simulink model "acc"  (R2021b)
settings: Solver=FixedStepAuto  StartTime=0.0  StopTime=206  FixedStep=0.0005  RelTol=1e-3
values from neighbouring files (symbols this model uses):
  Leftdis_PV_switch = 2    [acc_plot_backup.m]
  s_path = [0 1.10508939428 2.2141958029 3.32141571172 4.42705301151 5.53154548532 6.63517443471 7.73808041313 8.84055018688 9.94289959674 11.0453539299 12.1480581097 ... (1001 elements, 1001x1)]    [200_100radius.mat]    (also in LV_Clothoid_S_Turn_path.mat = [0 0.966832089581 1.93621320584 2.90214024471 3.86476766313 ; NEDC_path.mat = [0 0.414605943146 0.832514087334 1.25401518562 1.68216660344; Straight_East_into_curve.mat = [0 1.65770560069 3.32192925577 4.98420060507 6.64484613518 8; acc_plot_backup.m = Station_HV_m)
  X_path = [0 1.10508939428 2.2141958029 3.32141571172 4.42705301151 5.53154548532 6.63517443471 7.73808041313 8.84055018688 9.94289959674 11.0453539299 12.1480581097 ... (1001 elements, 1001x1)]    [200_100radius.mat]    (also in LV_Clothoid_S_Turn_path.mat = [-10 -9.03316791042 -8.06378679416 -7.09785975529 -6.1352323; NEDC_path.mat = [0 0.414605943146 0.832514087334 1.25401518562 1.68216660344; Straight_East_into_curve.mat = [0 1.65770560069 3.32192925577 4.98420060507 6.64484613518 8; acc_plot_backup.m = X_HV_m)
  Y_path = [0 -1.70364610795e-18 -7.41532896709e-18 1.46822109542e-17 4.74557362791e-17 6.12980216762e-17 9.25043977736e-17 1.24088240159e-16 1.5099156923e-16 1.7058517853e-16 1.90629227614e-16 2.09673434424e-16 ... (1001 elements, 1001x1)]    [200_100radius.mat]    (also in LV_Clothoid_S_Turn_path.mat = [0 -8.46153035536e-19 5.07382551045e-18 2.07356032218e-17 3.; NEDC_path.mat = [0 -3.50680326162e-18 -2.14111304971e-18 3.38197671014e-18 3; Straight_East_into_curve.mat = [0 1.29197709199e-18 2.81882429322e-18 3.49020462564e-17 6.7; acc_plot_backup.m = Y_HV_m)
undefined symbols (not defined in the file or in its folder): C_TICK_TIME_S, ENUM_ACCSTATE_DISABLED, ENUM_ACCSTATE_OFF, ENUM_ACCSTATE_STANDBY, FALSE, KVDI_ACCLongPressTime_ms, KVDI_ACCMaxActSpeed_kph, KVDI_ACCSetSpdIntial_kph, KVDI_ACCSpdLargeChange_kph, KVDI_LongPressConTime_ms, ONE_FLOAT, ONE_INT, R, Rw, T, TRUE, ZERO_FLOAT, ZERO_INT
libraries: simulink x16, dspstat3 x4, simulink_extras x2, Solver_SF x1
(part 3 of 4)

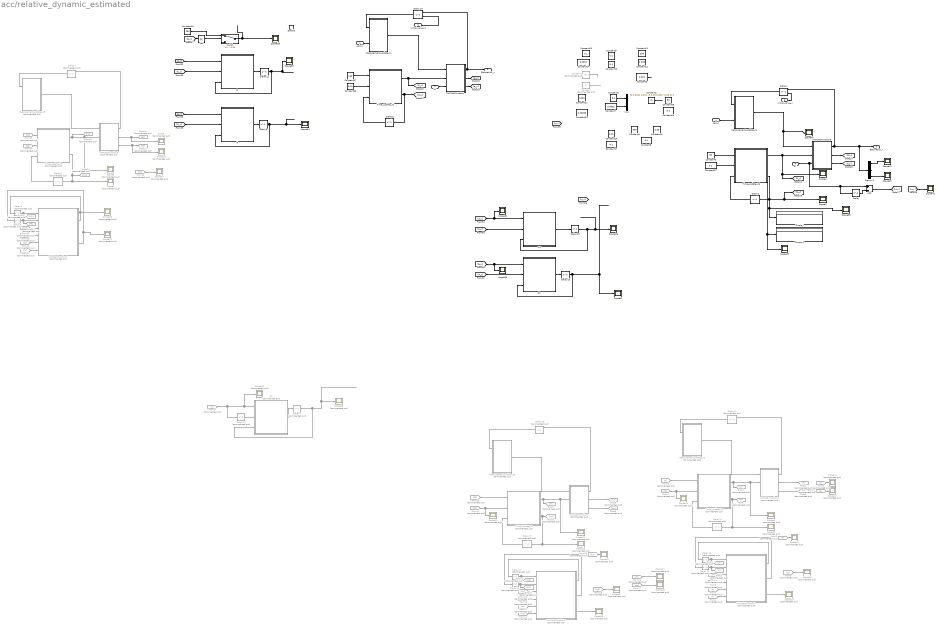
== system acc/relative_dynamic_estimated ==
  Jerk_X : Inport
  RX : Inport  Port=2
  Initial_value_X : Inport  Port=3
  Jerk_Y : Inport  Port=4
  RY : Inport  Port=5
  Initial_value_Y : Inport  Port=6
  Enable : EnablePort
  Abs : Abs
  Add : Sum  Inputs=+-
  Constant : Constant  Commented=on  Value=R
  Constant1 : Constant  Commented=on  Value=Rw
  Constant{4..5,9..10,13,17,22,24} (8 alike) : Constant  Value=0.1
  Constant11 : Constant  Value=200
  Constant12 : Constant  Value=0.005
  Constant14 : Constant  Value=0.0001
  Constant15 : Constant  Value=0.05
  Constant16 : Constant  Value=300
  Constant19 : Constant  Value=0.01
  Constant2 : Constant  Value=[0 0.0001 0.0017;0.0001 0.0025 0.05;0.0017 0.05 1]*1
  Constant20 : Constant  Value=0.00005
  Constant21 : Constant  Value=1000
  Constant25 : Constant  Value=50
  Constant26 : Constant  Value=0.01
  Constant27 : Constant  Value=100
  Constant3 : Constant  Value=0.001
  Constant6 : Constant  Value=50
  Constant7 : Constant  Value=0.0001
  Constant8 : Constant  Value=500
  Delay : Delay  DelayLength=1
  Delay1 : Delay  DelayLength=1  InitialConditionSource=Input port  InitialCondition=[0;0;0]  SampleTime=T
      settings: InputPortMap=u0,p4
  Delay10 : Delay  DelayLength=1  InitialConditionSource=Input port  InitialCondition=[0;0;0]  SampleTime=T
      settings: InputPortMap=u0,p4
  Delay11 : Delay  Commented=on  DelayLength=1  InitialConditionSource=Input port  InitialCondition=[0;0;0]  SampleTime=T
      settings: InputPortMap=u0,p4
  Delay12 : Delay  Commented=on  DelayLength=1  InitialCondition=[0 0 0;0 0 0.004;0 0.004 0.8]*0.001  SampleTime=T
  Delay13 : Delay  Commented=on  DelayLength=1  InitialCondition=0.001  SampleTime=T
  Delay14 : Delay  Commented=on  DelayLength=1  InitialCondition=[1 0 0;0 1 0;0 0 1]  SampleTime=T
  Delay15 : Delay  Commented=on  DelayLength=1  InitialConditionSource=Input port  InitialCondition=[0;0;0]  SampleTime=T
      settings: InputPortMap=u0,p4
  Delay16 : Delay  Commented=on  DelayLength=1  InitialCondition=0
  Delay17 : Delay  Commented=on  DelayLength=1  InitialCondition=[0 0 0;0 0 0.004;0 0.004 0.8]*0.01  SampleTime=T
  Delay18 : Delay  Commented=on  DelayLength=1  InitialCondition=0.001  SampleTime=T
  Delay19 : Delay  Commented=on  DelayLength=1  InitialCondition=[1 0 0;0 1 0;0 0 1]  SampleTime=T
  Delay2 : Delay  DelayLength=1  InitialCondition=[1 0 0;0 1 0;0 0 1]  SampleTime=T
  Delay21 : Delay  DelayLength=1  InitialCondition=[0 0.0001 0.0017;0.0001 0.0025 0.05;0.0017 0.05 1]
  Delay22 : Delay  DelayLength=1  InitialCondition=0.001
  Delay23 : Delay  DelayLength=1  InitialCondition=[0 0.0001 0.0017;0.0001 0.0025 0.05;0.0017 0.05 1]*1e-5
  Delay3 : Delay  Commented=on  DelayLength=1  InitialCondition=[0 0 0;0 0 0.003;0 0.003 0.005]  SampleTime=T
  Delay4 : Delay  Commented=on  DelayLength=1  InitialConditionSource=Input port  InitialCondition=[0;0;0]  SampleTime=T
      settings: InputPortMap=u0,p4
  Delay5 : Delay  Commented=on  DelayLength=1  InitialCondition=0.001  SampleTime=T
  Delay6 : Delay  Commented=on  DelayLength=1  InitialCondition=[1 0 0;0 1 0;0 0 1]  SampleTime=T
  Delay7 : Delay  Commented=on  DelayLength=1  InitialCondition=0.1
  Delay8 : Delay  DelayLength=1  InitialCondition=0.1
  Delay9 : Delay  DelayLength=1  InitialCondition=[1 0 0;0 1 0;0 0 1]  SampleTime=T
  Demux1 : Demux  Outputs=3
  Display : Display
  Display1 : Display
  From : From  Commented=on  GotoTag=M
  From1 : From  Commented=on  GotoTag=K
  From10 : From  Commented=on  GotoTag=MM
  From11 : From  Commented=on  GotoTag=KK
  From12 : From  Commented=on  GotoTag=dd
  From13 : From  Commented=on  GotoTag=ee
  From14 : From  Commented=on  GotoTag=QQ
  From15 : From  Commented=on  GotoTag=RR
  From16 : From  Commented=on  GotoTag=dd
  From17 : From  Commented=on  GotoTag=ee
  From18 : From  Commented=on  GotoTag=RR
  From19 : From  Commented=on  GotoTag=QQ
  From2 : From  Commented=on  GotoTag=d
  From20 : From  Commented=on  GotoTag=MM
  From21 : From  Commented=on  GotoTag=KK
  From22 : From  Commented=on  GotoTag=dd
  From23 : From  Commented=on  GotoTag=ee
  From24 : From  Commented=on  GotoTag=QQ
  From25 : From  Commented=on  GotoTag=RR
  From26 : From  Commented=on  GotoTag=KK
  From27 : From  Commented=on  GotoTag=d
  From3 : From  Commented=on  GotoTag=e
  From4 : From  Commented=on  GotoTag=Q
  From5 : From  Commented=on  GotoTag=R
  From6 : From  Commented=on  GotoTag=d
  From7 : From  Commented=on  GotoTag=e
  From8 : From  Commented=on  GotoTag=R
  From9 : From  Commented=on  GotoTag=Q
  Goto : Goto  Commented=on  GotoTag=M
  Goto1 : Goto  Commented=on  GotoTag=K
  Goto10 : Goto  Commented=on  GotoTag=QQ
  Goto11 : Goto  Commented=on  GotoTag=RR
  Goto12 : Goto  Commented=on  GotoTag=QQ
  Goto13 : Goto  Commented=on  GotoTag=RR
  Goto14 : Goto  Commented=on  GotoTag=MM
  Goto15 : Goto  Commented=on  GotoTag=KK
  Goto16 : Goto  Commented=on  GotoTag=dd
  Goto17 : Goto  Commented=on  GotoTag=ee
  Goto2 : Goto  Commented=on  GotoTag=d
  Goto3 : Goto  Commented=on  GotoTag=e
  Goto4 : Goto  Commented=on  GotoTag=Q
  Goto5 : Goto  Commented=on  GotoTag=R
  Goto6 : Goto  Commented=on  GotoTag=MM
  Goto7 : Goto  Commented=on  GotoTag=KK
  Goto8 : Goto  Commented=on  GotoTag=dd
  Goto9 : Goto  Commented=on  GotoTag=ee
  MATLAB Function : MATLAB Function  TreatAsAtomicUnit=on
  MATLAB Function1 : MATLAB Function  Commented=on  TreatAsAtomicUnit=on
  MATLAB Function2 : MATLAB Function  Commented=on  TreatAsAtomicUnit=on
  MATLAB Function3 : MATLAB Function  Commented=on  TreatAsAtomicUnit=on
  MATLAB Function4 : MATLAB Function  Commented=on  TreatAsAtomicUnit=on
  MATLAB Function5 : MATLAB Function  TreatAsAtomicUnit=on
  MATLAB Function6 : MATLAB Function  Commented=on  TreatAsAtomicUnit=on
  MATLAB Function7 : MATLAB Function  Commented=on  TreatAsAtomicUnit=on
  Measurement_update_X1 : MATLAB Function  TreatAsAtomicUnit=on
  Measurement_update_X2 : MATLAB Function  Commented=on  TreatAsAtomicUnit=on
  Measurement_update_X3 : MATLAB Function  Commented=on  TreatAsAtomicUnit=on
  Measurement_update_X4 : MATLAB Function  TreatAsAtomicUnit=on
  Measurement_update_X5 : MATLAB Function  Commented=on  TreatAsAtomicUnit=on
  Mux : Mux  Inputs=2
  Q : MATLAB Function  TreatAsAtomicUnit=on
  Q1 : MATLAB Function  Commented=on  TreatAsAtomicUnit=on
  Q2 : MATLAB Function  TreatAsAtomicUnit=on
  R : MATLAB Function  TreatAsAtomicUnit=on
  R2 : MATLAB Function  TreatAsAtomicUnit=on
  Scope{,6..28,30} (25 alike) : Scope  Commented=on
  Scope{1..2,5,29,31,34..43} (15 alike) : Scope
  Switch : Switch  Criteria=u2 > Threshold  Threshold=0.04
  Time_update_X1 : MATLAB Function  TreatAsAtomicUnit=on
  Time_update_X2 : MATLAB Function  Commented=on  TreatAsAtomicUnit=on
  Time_update_X3 : MATLAB Function  Commented=on  TreatAsAtomicUnit=on
  Time_update_X5 : MATLAB Function  Commented=on  TreatAsAtomicUnit=on
  Time_update_X6 : MATLAB Function  TreatAsAtomicUnit=on
  Estimation_X : Outport  VectorParamsAs1DForOutWhenUnconnected=off
  Estimation_Y : Outport  Port=2  VectorParamsAs1DForOutWhenUnconnected=off
  wires:
  MATLAB Function/3(e) -> [e_x]
  MATLAB Function/2(d) -> [d_x]
  Constant27/1 -> Time_update_X1/1(Q)
  Constant26/1 -> Time_update_X1/2(R)
  Abs/1 -> Switch/2
  [d_x] -> Abs/1
  Constant16/1 -> Switch/1
  Switch/1 -> Scope39/1
  Constant22/1 -> Time_update_X6/2(R)
  Constant6/1 -> Time_update_X6/1(Q)
  Demux1/3 -> Scope43/1
  Demux1/1 -> Scope42/1
  [yyy] -> Scope41/1
  Delay/1 -> Add/2
  Add/1 -> [yyy]
  Delay22/1 -> Scope5/1, R2/3(R1)
  Constant7/1 -> Mux/2
  Constant4/1 -> Mux/1
  Demux1/2 -> ?
  Delay23/1 -> Scope36/1, Q2/3(Q1)
  Time_update_X6/2(P) -> Display1/1, Scope37/1
  Constant3/1 -> ?
  Constant2/1 -> ?
  Q2/1(Q) -> Delay23/1
  Constant1/1 -> ?
  Constant/1 -> ?
  MATLAB Function5/3(e) -> [e_y]
  MATLAB Function5/2(d) -> [d_y]
  [d_y] -> Q2/1(d), Scope31/1
  [K_y] -> Q2/2(K)
  R2/1(R) -> Delay22/1
  [M_y] -> R2/2(M)
  [e_y] -> R2/1(e), Scope29/1
  Q1/1(Rw) -> Delay7/1
  From27/1 -> Q1/1(d), Scope30/1, Delay16/1
  Delay7/1 -> Scope28/1, Q1/3(Rw1)
  Delay16/1 -> Q1/2(dx)
  Delay21/1 -> Q/3(Q1), Scope35/1
  Q/1(Q) -> Delay21/1
  [K_x] -> Q/2(K)
  [d_x] -> Q/1(d)
  [M_x] -> R/2(M)
  R/1(R) -> Delay8/1
  [e_x] -> R/1(e)
  Delay8/1 -> R/3(R1), Scope34/1
  RX/1 -> MATLAB Function/3(y)
  From26/1 -> Scope27/1
  Initial_value_X/1 -> Delay10/2
  Delay4/1 -> Measurement_update_X5/1(X_e)
  MATLAB Function6/1(X_e) -> Delay4/1
  Measurement_update_X5/1(X_b) -> MATLAB Function6/1(X_b)
  Time_update_X5/2(M2) -> Scope7/1, Delay6/1, Goto14/1
  From22/1 -> MATLAB Function7/5(d)
  Delay6/1 -> Time_update_X5/3(M)
  Time_update_X5/1(K) -> MATLAB Function6/2(K), Scope6/1, Goto15/1
  From21/1 -> MATLAB Function7/6(K)
  From20/1 -> MATLAB Function7/3(M)
  MATLAB Function7/2(R2) -> Delay5/1, Scope26/1
  MATLAB Function6/3(e) -> Goto17/1, Scope24/1
  From24/1 -> Time_update_X5/2(Q)
  From25/1 -> Time_update_X5/1(R)
  MATLAB Function7/1(Q2) -> Scope25/1, Delay3/1
  From23/1 -> MATLAB Function7/4(e)
  Delay5/1 -> Goto13/1, MATLAB Function7/2(R)
  Delay3/1 -> Goto12/1, MATLAB Function7/1(Q)
  MATLAB Function6/2(d) -> Goto16/1, Scope/1
  RY/1 -> MATLAB Function5/3(y), Delay/1, Add/1
  Initial_value_Y/1 -> Delay1/2
  Measurement_update_X4/1(X_b) -> MATLAB Function5/1(X_b), Scope40/1
  MATLAB Function5/1(X_e) -> Delay1/1, Estimation_Y/1, Demux1/1
  Delay1/1 -> Measurement_update_X4/1(X_e)
  Time_update_X6/1(K) -> Scope1/1, [K_y], MATLAB Function5/2(K)
  Time_update_X6/3(M2) -> Delay2/1, Scope2/1, [M_y], Display/1, Scope38/1
  Delay2/1 -> Time_update_X6/3(M)
  Jerk_Y/1 -> Measurement_update_X4/2(u)
  Jerk_X/1 -> Measurement_update_X1/2(u)
  MATLAB Function3/2(d) -> Goto8/1
  Delay17/1 -> MATLAB Function4/1(Q), Goto10/1
  Time_update_X3/1(K) -> MATLAB Function3/2(K), Scope22/1, Goto7/1
  From13/1 -> MATLAB Function4/4(e)
  From15/1 -> Time_update_X3/1(R)
  From19/1 -> Scope21/1
  MATLAB Function4/1(Q2) -> Delay17/1
  Delay18/1 -> MATLAB Function4/2(R), Goto11/1
  From10/1 -> MATLAB Function4/3(M)
  MATLAB Function4/2(R2) -> Delay18/1
  Delay15/1 -> Measurement_update_X3/1(X_e)
  From11/1 -> MATLAB Function4/6(K)
  Delay19/1 -> Time_update_X3/3(M)
  From12/1 -> MATLAB Function4/5(d)
  From17/1 -> Scope18/1
  From18/1 -> Scope19/1
  From16/1 -> Scope17/1
  MATLAB Function3/3(e) -> Goto9/1
  Time_update_X3/2(M2) -> Goto6/1, Delay19/1, Scope23/1
  Measurement_update_X3/1(X_b) -> MATLAB Function3/1(X_b)
  From14/1 -> Time_update_X3/2(Q), Scope16/1
  MATLAB Function3/1(X_e) -> Delay15/1
  MATLAB Function4/3(G) -> Scope20/1
  From9/1 -> Scope15/1
  MATLAB Function2/3(G) -> Scope14/1
  From8/1 -> Scope13/1
  From7/1 -> Scope12/1
  From6/1 -> Scope11/1
  From4/1 -> Time_update_X2/2(Q), Scope10/1
  MATLAB Function2/1(Q2) -> Delay12/1
  Time_update_X2/2(M2) -> Goto/1, Delay14/1, Scope9/1
  From1/1 -> MATLAB Function2/6(K)
  Delay13/1 -> MATLAB Function2/2(R), Goto5/1
  Delay14/1 -> Time_update_X2/3(M)
  Time_update_X2/1(K) -> MATLAB Function1/2(K), Scope8/1, Goto1/1
  Delay11/1 -> Measurement_update_X2/1(X_e)
  Measurement_update_X2/1(X_b) -> MATLAB Function1/1(X_b)
  MATLAB Function1/1(X_e) -> Delay11/1
  MATLAB Function1/2(d) -> Goto2/1
  From2/1 -> MATLAB Function2/5(d)
  From5/1 -> Time_update_X2/1(R)
  MATLAB Function1/3(e) -> Goto3/1
  MATLAB Function2/2(R2) -> Delay13/1
  From/1 -> MATLAB Function2/3(M)
  From3/1 -> MATLAB Function2/4(e)
  Delay12/1 -> MATLAB Function2/1(Q), Goto4/1
  MATLAB Function/1(X_e) -> Delay10/1, Estimation_X/1
  Time_update_X1/2(M2) -> Delay9/1, [M_x]
  Measurement_update_X1/1(X_b) -> MATLAB Function/1(X_b)
  Delay9/1 -> Time_update_X1/3(M)
  Delay10/1 -> Measurement_update_X1/1(X_e)
  Time_update_X1/1(K) -> MATLAB Function/2(K), [K_x]

== system acc/rolling_avg ==
  note: new_average = [ (sample_interval)/(sample_interval + time_constant) ] * (new_value - old_ave) + old_ave
  note: - (FK_TMR/TC)
      |                                    f  =  1  -  e
      |
      |       Where "f" is called the filter constant in the difference equation:
      |
      |                    new_average = f * new_value + (1 - f) * old_average
  note: Using the first two terms of the series expansion:
      |
      |                     x                     x2
      |                                e   =  1  +  x  +  --  + ......
      |                                           2!
      |
      |       Simplifying, the exponential "f" becomes:
      |
      |                  - (FK_TMR/TC)              1
      |           f  =  1  -  e                    =  1  -  -------------  =  . . .
      |                                                    (FK_TMR/TC)
      |                           e
      |
      |                              1                      1
      |          f  =  1  -  ---------------------------------  =    ------------------- .
      |                                  1 + (FK_TMR / TC)       1 + (TC / FK_TMR)
  new_value : Inport
  old_ave : Inport  Port=2
  delta_t : Inport  Port=3
  tc : Inport  Port=4
  Divide : Product  Inputs=*/
  IC : UnitDelay  Tag=struct('comment',struct('text','','placement',1),'logdata',struct('maxnumvals',inf,'plotchannels',[],'stepsize',0,'downsampling',1,'loggingmode',3,'channels',1),'output',struct('width',1,'name','$S_$B','unit','','type','Int16','offset',0,'max',NaN,'min',NaN,'freeze',1,'lsb',1,'arb',0,'class','default','address','','description','','autoscalingmode',1,'lowerheadroom',1,'upperheadroom',1,'headroomunit','bit','checkmin',0,'checkmax',0,'show',0,'initial','2'),'state',0,'dt','-1','date',731455.586925799)  InitialCondition=1  SampleTime=0.1  HasFrameUpgradeWarning=on
  Interval Test : simulink/Logic and Bit Operations/Interval Test  IntervalClosedRight=on  uplimit=0.00001  IntervalClosedLeft=on  lowlimit=-0.00001  OutDataTypeStr=boolean
  Logical Operator : Logic  Operator=NOT  AllPortsSameDT=off  OutDataTypeStr=boolean
  Product_tmp1 : Product  Tag=struct('comment',struct('text','','placement',1),'logdata',struct('maxnumvals',inf,'plotchannels',[],'stepsize',0,'downsampling',1,'loggingmode',3,'channels',1),'output',struct('width',1,'name','$S_$B','unit','','type','Int32Bin15','offset',0,'max',65535,'min',-65536,'freeze',1,'lsb',2^-15,'arb',0,'class','default','address','','description','','autoscalingmode',1,'lowerheadroom',1,'upperheadroom',1,'headroomunit','bit','checkmin',0,'checkmax',0,'show',0),'inputs','**','exceptionhandling',1,'date',731455.58640515)  Inputs=**  InputSameDT=on  RndMeth=Zero  OutDataTypeStr=Inherit: Same as first input
  Sum : Sum  Tag=struct('comment',struct('text','','placement',1),'logdata',struct('maxnumvals',inf,'plotchannels',[],'stepsize',0,'downsampling',1,'loggingmode',3,'channels',1),'output',struct('width',1,'name','$S_$B','unit','','type','Int32Bin15','offset',0,'max',65535,'min',-65536,'freeze',1,'lsb',2^-15,'arb',0,'class','default','address','','description','','autoscalingmode',1,'lowerheadroom',1,'upperheadroom',1,'headroomunit','bit','checkmin',0,'checkmax',0,'show',0),'inputs','-+','date',731455.586330463)  Inputs=-+  InputSameDT=on  OutDataTypeStr=Inherit: Same as first input
  Sum1 : Sum  Tag=struct('comment',struct('text','','placement',1),'logdata',struct('maxnumvals',inf,'plotchannels',[],'stepsize',0,'downsampling',1,'loggingmode',3,'channels',1),'output',struct('width',1,'name','$S_$B','unit','','type','Int32Bin15','offset',0,'max',65535,'min',-65536,'freeze',1,'lsb',2^-15,'arb',0,'class','default','address','','description','','autoscalingmode',1,'lowerheadroom',1,'upperheadroom',1,'headroomunit','bit','checkmin',0,'checkmax',0,'show',0),'inputs','++','date',731455.58628235)  InputSameDT=on  OutDataTypeStr=Inherit: Same as first input
  Sum2 : Sum  Tag=struct('comment',struct('text','','placement',1),'logdata',struct('maxnumvals',inf,'plotchannels',[],'stepsize',0,'downsampling',1,'loggingmode',3,'channels',1),'output',struct('width',1,'name','$S_$B','unit','','type','Int32Bin15','offset',0,'max',65535,'min',-65536,'freeze',1,'lsb',2^-15,'arb',0,'class','default','address','','description','','autoscalingmode',1,'lowerheadroom',1,'upperheadroom',1,'headroomunit','bit','checkmin',0,'checkmax',0,'show',0),'inputs','++','date',731455.586506424)  InputSameDT=on  OutDataTypeStr=Inherit: Same as first input
  Switch : Switch  Criteria=u2 ~= 0
  Switch1 : Switch  Tag=struct('comment',struct('text','','placement',1),'logdata',struct('maxnumvals',inf,'plotchannels',[],'stepsize',0,'downsampling',1,'loggingmode',3,'channels',1),'output',struct('width',1,'name','$S_$B','unit','','type','Int32Bin15','offset',0,'max',65535,'min',-65536,'freeze',1,'lsb',2^-15,'arb',0,'class','default','address','','description','','autoscalingmode',1,'lowerheadroom',1,'upperheadroom',1,'headroomunit','bit','checkmin',0,'checkmax',0,'show',0),'threshold',struct('width',1,'name','$S_$B_threshold','unit','','type','Int16','offset',0,'max',NaN,'min',NaN,'freeze',1,'lsb',1,'arb',0,'class','default','address','','description','','value','1','scalar',0),'date',731455.58657044)  Threshold=0.5  InputSameDT=on
  zero : Constant  Tag=struct('comment',struct('text','','placement',1),'output',struct('width',1,'name','$S_$B','unit','','type','Int16','offset',0,'max',NaN,'min',NaN,'freeze',1,'lsb',1,'arb',0,'class','default','address','','description','','value','0','tolerance',1,'show',0),'date',731455.58675544)  Value=0  OutDataTypeStr=Inherit: Inherit via back propagation
  zero1 : Constant  Tag=struct('comment',struct('text','','placement',1),'output',struct('width',1,'name','$S_$B','unit','','type','Int16','offset',0,'max',NaN,'min',NaN,'freeze',1,'lsb',1,'arb',0,'class','default','address','','description','','value','0','tolerance',1,'show',0),'date',731455.58675544)  Value=0  OutDataTypeStr=Inherit: Inherit via back propagation
  new_ave : Outport
  wires:
  Switch/1 -> Sum2/2
  Product_tmp1/1 -> Divide/1
  [new_value] -> Switch1/1
  Sum2/1 -> Switch1/3  "new_ave"
  new_value/1 -> [new_value], Sum/2  "new_value"
  Switch1/1 -> new_ave/1  "new_ave"
  Sum/1 -> Product_tmp1/1
  tc/1 -> Sum1/2
  delta_t/1 -> Sum1/1, Product_tmp1/2  "delta_t"
  zero/1 -> IC/1
  old_ave/1 -> Sum/1, Sum2/1  "old_ave"
  Sum1/1 -> Interval Test/1, Divide/2
  zero1/1 -> Switch/3
  Interval Test/1 -> Logical Operator/1
  Divide/1 -> Switch/1
  Logical Operator/1 -> Switch/2
  IC/1 -> Switch1/2

== system acc/velocity_apr5 ==
  velocity_b : Inport
  Abs : Abs
  Constant1 : Constant  Value=0
  Switch : Switch  Criteria=u2 > Threshold  Threshold=0.1
  velocity_a : Outport  VectorParamsAs1DForOutWhenUnconnected=off
  wires:
  Abs/1 -> Switch/2
  Constant1/1 -> Switch/3
  velocity_b/1 -> Switch/1, Abs/1
  Switch/1 -> velocity_a/1

== system acc/Cut-in strategy/Subsystem8 ==
  TTC : Inport
  Mode : Inport  Port=2
  Constant1 : Constant  Value=0
  Gain : Gain  Gain=5
  Switch : Switch  Criteria=u2 ~= 0
  tau : Outport
  wires:
  Constant1/1 -> Switch/3
  TTC/1 -> Gain/1
  Switch/1 -> tau/1
  Mode/1 -> Switch/2
  Gain/1 -> Switch/1

== system acc/Smooth Switch/Subsystem ==
  TTC : Inport
  Mode : Inport  Port=2
  1-D Lookup Table : Lookup_n-D  NumberOfTableDimensions=1  BreakpointsForDimension1=[0 2 10]  Table=[0.05 0.05 0.5]  InternalRulePriority=Speed  RndMeth=Simplest  InputSameDT=on
  Constant1 : Constant  Value=0.5
  Constant2 : Constant
  Constant3 : Constant  Value=0.01
  Switch : Switch  Criteria=u2 ~= 0
  tau : Outport
  wires:
  Constant1/1 -> Switch/1
  Switch/1 -> tau/1
  Mode/1 -> Switch/2
  TTC/1 -> 1-D Lookup Table/1
  1-D Lookup Table/1 -> Switch/3

== system acc/Subsystem/cut_off5 ==
  sign : Inport
  in : Inport  Port=2
  Delay : Delay  DelayLength=1  InitialConditionSource=Input port
      settings: InputPortMap=u0,p4
  Switch16 : Switch  Criteria=u2 ~= 0
  Out : Outport  VectorParamsAs1DForOutWhenUnconnected=off
  wires:
  in/1 -> Delay/2, Switch16/3
  sign/1 -> Switch16/2
  Switch16/1 -> Out/1, Delay/1
  Delay/1 -> Switch16/1

== system acc/Subsystem2/Smooth_Switch1 ==
  In1 : Inport
  Add : Sum
  Add1 : Sum  Inputs=+-
  Constant : Constant  Value=T/tau
  Constant1 : Constant
  Product : Product
  Product1 : Product
  Unit Delay : UnitDelay  InitialCondition=IC  SampleTime=T  HasFrameUpgradeWarning=on
  Out1 : Outport
  wires:
  Constant1/1 -> Add1/1
  Constant/1 -> Add1/2, Product1/2
  Add1/1 -> Product/1
  In1/1 -> Product1/1
  Product/1 -> Add/2
  Unit Delay/1 -> Product/2, Out1/1
  Add/1 -> Unit Delay/1
  Product1/1 -> Add/1

== system acc/Subsystem4/rolling_avg1 ==
  note: Using the first two terms of the series expansion:
      |
      |                     x                     x2
      |                                e   =  1  +  x  +  --  + ......
      |                                           2!
      |
      |       Simplifying, the exponential "f" becomes:
      |
      |                  - (FK_TMR/TC)              1
      |           f  =  1  -  e                    =  1  -  -------------  =  . . .
      |                                                    (FK_TMR/TC)
      |                           e
      |
      |                              1                      1
      |          f  =  1  -  ---------------------------------  =    ------------------- .
      |                                  1 + (FK_TMR / TC)       1 + (TC / FK_TMR)
  note: - (FK_TMR/TC)
      |                                    f  =  1  -  e
      |
      |       Where "f" is called the filter constant in the difference equation:
      |
      |                    new_average = f * new_value + (1 - f) * old_average
  note: new_average = [ (sample_interval)/(sample_interval + time_constant) ] * (new_value - old_ave) + old_ave
  new_value : Inport
  old_ave : Inport  Port=2
  delta_t : Inport  Port=3
  tc : Inport  Port=4
  Divide : Product  Inputs=*/
  IC : UnitDelay  Tag=struct('comment',struct('text','','placement',1),'logdata',struct('maxnumvals',inf,'plotchannels',[],'stepsize',0,'downsampling',1,'loggingmode',3,'channels',1),'output',struct('width',1,'name','$S_$B','unit','','type','Int16','offset',0,'max',NaN,'min',NaN,'freeze',1,'lsb',1,'arb',0,'class','default','address','','description','','autoscalingmode',1,'lowerheadroom',1,'upperheadroom',1,'headroomunit','bit','checkmin',0,'checkmax',0,'show',0,'initial','2'),'state',0,'dt','-1','date',731455.586925799)  InitialCondition=1  SampleTime=0.1  HasFrameUpgradeWarning=on
  Interval Test : simulink/Logic and Bit Operations/Interval Test  IntervalClosedRight=on  uplimit=0.00001  IntervalClosedLeft=on  lowlimit=-0.00001  OutDataTypeStr=boolean
  Logical Operator : Logic  Operator=NOT  AllPortsSameDT=off  OutDataTypeStr=boolean
  Product_tmp1 : Product  Tag=struct('comment',struct('text','','placement',1),'logdata',struct('maxnumvals',inf,'plotchannels',[],'stepsize',0,'downsampling',1,'loggingmode',3,'channels',1),'output',struct('width',1,'name','$S_$B','unit','','type','Int32Bin15','offset',0,'max',65535,'min',-65536,'freeze',1,'lsb',2^-15,'arb',0,'class','default','address','','description','','autoscalingmode',1,'lowerheadroom',1,'upperheadroom',1,'headroomunit','bit','checkmin',0,'checkmax',0,'show',0),'inputs','**','exceptionhandling',1,'date',731455.58640515)  Inputs=**  InputSameDT=on  RndMeth=Zero  OutDataTypeStr=Inherit: Same as first input
  Sum : Sum  Tag=struct('comment',struct('text','','placement',1),'logdata',struct('maxnumvals',inf,'plotchannels',[],'stepsize',0,'downsampling',1,'loggingmode',3,'channels',1),'output',struct('width',1,'name','$S_$B','unit','','type','Int32Bin15','offset',0,'max',65535,'min',-65536,'freeze',1,'lsb',2^-15,'arb',0,'class','default','address','','description','','autoscalingmode',1,'lowerheadroom',1,'upperheadroom',1,'headroomunit','bit','checkmin',0,'checkmax',0,'show',0),'inputs','-+','date',731455.586330463)  Inputs=-+  InputSameDT=on  OutDataTypeStr=Inherit: Same as first input
  Sum1 : Sum  Tag=struct('comment',struct('text','','placement',1),'logdata',struct('maxnumvals',inf,'plotchannels',[],'stepsize',0,'downsampling',1,'loggingmode',3,'channels',1),'output',struct('width',1,'name','$S_$B','unit','','type','Int32Bin15','offset',0,'max',65535,'min',-65536,'freeze',1,'lsb',2^-15,'arb',0,'class','default','address','','description','','autoscalingmode',1,'lowerheadroom',1,'upperheadroom',1,'headroomunit','bit','checkmin',0,'checkmax',0,'show',0),'inputs','++','date',731455.58628235)  InputSameDT=on  OutDataTypeStr=Inherit: Same as first input
  Sum2 : Sum  Tag=struct('comment',struct('text','','placement',1),'logdata',struct('maxnumvals',inf,'plotchannels',[],'stepsize',0,'downsampling',1,'loggingmode',3,'channels',1),'output',struct('width',1,'name','$S_$B','unit','','type','Int32Bin15','offset',0,'max',65535,'min',-65536,'freeze',1,'lsb',2^-15,'arb',0,'class','default','address','','description','','autoscalingmode',1,'lowerheadroom',1,'upperheadroom',1,'headroomunit','bit','checkmin',0,'checkmax',0,'show',0),'inputs','++','date',731455.586506424)  InputSameDT=on  OutDataTypeStr=Inherit: Same as first input
  Switch : Switch  Criteria=u2 ~= 0
  Switch1 : Switch  Tag=struct('comment',struct('text','','placement',1),'logdata',struct('maxnumvals',inf,'plotchannels',[],'stepsize',0,'downsampling',1,'loggingmode',3,'channels',1),'output',struct('width',1,'name','$S_$B','unit','','type','Int32Bin15','offset',0,'max',65535,'min',-65536,'freeze',1,'lsb',2^-15,'arb',0,'class','default','address','','description','','autoscalingmode',1,'lowerheadroom',1,'upperheadroom',1,'headroomunit','bit','checkmin',0,'checkmax',0,'show',0),'threshold',struct('width',1,'name','$S_$B_threshold','unit','','type','Int16','offset',0,'max',NaN,'min',NaN,'freeze',1,'lsb',1,'arb',0,'class','default','address','','description','','value','1','scalar',0),'date',731455.58657044)  Threshold=0.5  InputSameDT=on
  zero : Constant  Tag=struct('comment',struct('text','','placement',1),'output',struct('width',1,'name','$S_$B','unit','','type','Int16','offset',0,'max',NaN,'min',NaN,'freeze',1,'lsb',1,'arb',0,'class','default','address','','description','','value','0','tolerance',1,'show',0),'date',731455.58675544)  Value=0  OutDataTypeStr=Inherit: Inherit via back propagation
  zero1 : Constant  Tag=struct('comment',struct('text','','placement',1),'output',struct('width',1,'name','$S_$B','unit','','type','Int16','offset',0,'max',NaN,'min',NaN,'freeze',1,'lsb',1,'arb',0,'class','default','address','','description','','value','0','tolerance',1,'show',0),'date',731455.58675544)  Value=0  OutDataTypeStr=Inherit: Inherit via back propagation
  new_ave : Outport
  wires:
  IC/1 -> Switch1/2
  Logical Operator/1 -> Switch/2
  Divide/1 -> Switch/1
  Interval Test/1 -> Logical Operator/1
  zero1/1 -> Switch/3
  Sum1/1 -> Divide/2, Interval Test/1
  old_ave/1 -> Sum2/1, Sum/1  "old_ave"
  zero/1 -> IC/1
  delta_t/1 -> Product_tmp1/2, Sum1/1  "delta_t"
  tc/1 -> Sum1/2
  Sum/1 -> Product_tmp1/1
  Switch1/1 -> new_ave/1  "new_ave"
  new_value/1 -> Sum/2, [new_value]  "new_value"
  Sum2/1 -> Switch1/3  "new_ave"
  [new_value] -> Switch1/1
  Product_tmp1/1 -> Divide/1
  Switch/1 -> Sum2/2

== system acc/V_rel Estimation/Kalman filter ==
  cut_in_flg : Inport
  Jerk : Inport  Port=2
  S_rel : Inport  Port=3
  initial_value : Inport  Port=4
  Constant : Constant  Value=200  OutDataTypeStr=double
  Constant1 : Constant  Value=0.01  OutDataTypeStr=double
  Delay : Delay  DelayLength=1  InitialCondition=[1 0 0;0 1 0;0 0 1]  SampleTime=0.1
  Delay1 : Delay  DelayLength=1  InitialConditionSource=Input port  InitialCondition=[1;1;1]  ExternalReset=Rising  SampleTime=0.1
      settings: InputPortMap=u0,r5,p4
  Demux3 : Demux  Outputs=[1 1 1]
      settings: DisplayOption=none
  MATLAB Function2 : MATLAB Function  TreatAsAtomicUnit=on
  measurement update : MATLAB Function  TreatAsAtomicUnit=on
  time update : MATLAB Function  TreatAsAtomicUnit=on
  s_rel : Outport
  v_rel : Outport  Port=2
  a_rel : Outport  Port=3
  wires:
  S_rel/1 -> MATLAB Function2/3(Y)
  measurement update/1(X1) -> MATLAB Function2/1(X1)
  MATLAB Function2/1(X2) -> Demux3/1, Delay1/1
  Constant/1 -> time update/1(Q)
  initial_value/1 -> Delay1/3
  Delay/1 -> time update/3(M1)
  time update/2(M2) -> Delay/1
  Delay1/1 -> measurement update/1(X2)
  Constant1/1 -> time update/2(R)
  time update/1(K) -> MATLAB Function2/2(K)
  Demux3/1 -> s_rel/1
  Demux3/2 -> v_rel/1
  Demux3/3 -> a_rel/1
  Jerk/1 -> measurement update/2(u)
  cut_in_flg/1 -> Delay1/2

== system acc/cmd_limiter2/Smooth Switch ==
  smaller_cmd : Inport
  Mode : Inport  Port=2
  Larger_cmd : Inport  Port=3
  Add12 : Sum
  Add9 : Sum  Inputs=+-
  Constant49 : Constant
  Data Type Conversion : DataTypeConversion  OutDataTypeStr=double
  Delay : Delay  DelayLength=1  InitialConditionSource=Input port  SampleTime=0.1
      settings: InputPortMap=u0,p4
  MATLAB Function : MATLAB Function  TreatAsAtomicUnit=on
  Product1 : Product
  Product2 : Product
  Scope : Scope
  Subsystem : Subsystem
  ax_cmd : Outport
  wires:
  Product2/1 -> Add12/1
  smaller_cmd/1 -> Product2/1
  MATLAB Function/1(y) -> Scope/1, Product2/2, Add9/2, Delay/1
  Data Type Conversion/1 -> Delay/2, MATLAB Function/2(u)
  Constant49/1 -> Add9/1
  Product1/1 -> Add12/2
  Larger_cmd/1 -> Product1/2
  Add9/1 -> Product1/1
  Add12/1 -> ax_cmd/1
  Mode/1 -> Subsystem/1(In1), Data Type Conversion/1
  Delay/1 -> MATLAB Function/3(old_u)
  Subsystem/1(Out1) -> MATLAB Function/1(tau)

== system acc/cmd_limiter3/Smooth Switch ==
  smaller_cmd : Inport
  Mode : Inport  Port=2
  Larger_cmd : Inport  Port=3
  Add12 : Sum
  Add9 : Sum  Inputs=+-
  Constant49 : Constant
  Data Type Conversion : DataTypeConversion  OutDataTypeStr=double
  Delay : Delay  DelayLength=1  SampleTime=0.1
  MATLAB Function : MATLAB Function  TreatAsAtomicUnit=on
  Product1 : Product
  Product2 : Product
  Scope : Scope
  Subsystem : Subsystem
  ax_cmd : Outport
  wires:
  Subsystem/1(Out1) -> MATLAB Function/1(tau)
  Delay/1 -> MATLAB Function/3(old_u)
  Mode/1 -> Data Type Conversion/1, Subsystem/1(In1)
  Add12/1 -> ax_cmd/1
  Add9/1 -> Product1/1
  Larger_cmd/1 -> Product1/2
  Product1/1 -> Add12/2
  Constant49/1 -> Add9/1
  Data Type Conversion/1 -> MATLAB Function/2(u)
  MATLAB Function/1(y) -> Delay/1, Add9/2, Product2/2, Scope/1
  smaller_cmd/1 -> Product2/1
  Product2/1 -> Add12/1

== system acc/cmd_limiter2/Smooth Switch/Subsystem ==
  In1 : Inport
  Constant1 : Constant
  Constant2 : Constant
  Switch : Switch  Criteria=u2 ~= 0
  Out1 : Outport
  wires:
  Constant1/1 -> Switch/1
  Constant2/1 -> Switch/3
  Switch/1 -> Out1/1
  In1/1 -> Switch/2

== system acc/cmd_limiter3/Smooth Switch/Subsystem ==
  In1 : Inport
  Constant1 : Constant
  Constant2 : Constant
  Switch : Switch  Criteria=u2 ~= 0
  Out1 : Outport
  wires:
  In1/1 -> Switch/2
  Switch/1 -> Out1/1
  Constant2/1 -> Switch/3
  Constant1/1 -> Switch/1

== matlab function acc/MATLAB Function1 ==
  data: mode input; u output; Yref input; Vx input; ax input; D_rel input; V_rel input; ax_rel input; Qs input; Rs input; Y output
function [u,Y] = fcn(mode,Yref,Vx,ax,D_rel,V_rel,ax_rel,Qs,Rs)
%% Initialzization
T = 0.1;
tau = 0.3;
Np = 10;
Nc = 3;
%% TH Estimation
% Vx_TH = zeros(Np,1);
% 
% for i = 1:Np
%     t = i*0.1;
%     V_p = Vx+ax*t;
%     
%     if Vx-(5/3.6) < abs(1/3.6)
%         Vx_TH(i)=2+V_p*TH_ref;   % stop & go 
%     else
%         Vx_TH(i) = V_p*TH_ref;   % Track TH ref
%     end
% %     Vx_TH(i) = TH_ref*(Vx+ax*(i-1)*T);
%     
% end

%% Mode Selector && MPC
%Mode 1 = Speed control
%Mode 2 = TH and Stop&Go Control

A_rel = [1 T 0.5*T^2;
         0 1 T;
         0 0 1-T/tau];
% B = [1/6*T^3;0.5*T^2;T/tau];
B_rel = [0;0;T/tau];
C_rel = [1 0 0];

if mode == 1
    [m2,n2] = size(C_rel);
    h = zeros(Np,n2);
    F = zeros(Np,n2);
    h(1,:)=C_rel;
    F(1,:)=C_rel*A_rel;
    for j=2:Np
    h(j,:)=h(j-1,:)*A_rel; %Phi
    F(j,:)= F(j-1,:)*A_rel; 
    end
    v = h*B_rel;
    Phi_vx = zeros(Np,Nc);
    Phi_vx(:,1) = v;
    for k = 2:Nc
       Phi_vx(:,k) = [zeros(k-1,1);v(1:Np-k+1,1)]; %Toeplitz matrix
    end
    Q=Qs.*eye(Np); %Qw權重值=1;10
    R=Rs.*eye(Nc);%Rw權重值=0.07;1.5 ,0.07
    
    x_rel = [D_rel;V_rel;ax_rel];
    
    H = Phi_vx'*Q*Phi_vx+R;
    f = Phi_vx'*Q*(Yref-F*x_rel);
    U = inv(H)*f;
    u = (ax+ax_rel)-U(1);
%     if u > 0
%     u = min([u 2]);
%     else
%     u = max([-2 u]);
%     end
    Y=Yref(1);
else
    u=0;
    Y=0;
end
end

== matlab function acc/relative_dynamic_estimated/MATLAB Function5 ==
  data: X_b input; X_e output; K input; y input; d output; e output
function [X_e,d,e] = fcn(X_b,K,y)
H=[1 0 0];

X_e=X_b+K*(y-H*X_b);
d=y-H*X_b;
e=y-H*X_e;
end

== matlab function acc/relative_dynamic_estimated/Measurement_update_X4 ==
  data: X_e input; u input; X_b output
function X_b=fcn(X_e,u)
T=0.1;
F=[1 T 0.5*T^2;0 1 T;0 0 1];
G=[-1/6*T^3;-1/2*T^2;-T];

X_b=F*X_e+G*u;
end

== matlab function acc/V_rel Estimation/Kalman filter/MATLAB Function2 ==
  data: X1 input; X2 output; K input; Y input
function X2 = fcn(X1,K,Y)%Y=相對速度
H=[1 0 0];
X2=X1+K*(Y-H*X1);
end

== matlab function acc/V_rel Estimation/Kalman filter/measurement update ==
  data: X2 input; u input; X1 output
function X1 = fcn(X2,u)%u=jerk input
T=0.1;
F=[1 T 0.5*T^2;0 1 T;0 0 1];
G=[-1/6*T^3;-1/2*T^2;-T];
X1=F*X2+G*u;
end

== matlab function acc/relative_dynamic_estimated/MATLAB Function ==
  data: X_b input; X_e output; K input; y input; d output; e output
function [X_e,d,e] = fcn(X_b,K,y)
H=[1 0 0];

X_e=X_b+K*(y-H*X_b);
d=y-H*X_b;
e=y-H*X_e;
end

== matlab function acc/relative_dynamic_estimated/Q2 ==
  data: Q output; d input; K input; Q1 input
function Q  = fcn(d,K,Q1)
if abs(d) > 0.002
    Q=0.3*Q1+0.7*(K*d*d*K');
else
    Q=Q1;
end

end

== matlab function acc/V_rel Estimation/Kalman filter/time update ==
  data: Q input; K output; R input; M1 input; M2 output
function [K,M2] = fcn(Q,R,M1)
T=0.1;%sample time
F=[1 T 0.5*T^2;0 1 T;0 0 1];%system matrix
H=[1 0 0];%output matrix
G=[-(T^3)/6;-(T^2)/2;-T];%
%誤差斜方矩陣
P=M1-M1*H'*inv(H*M1*H'+R)*H*M1;
M2=F*P*F'+G*Q*G';
K=P*H'*inv(R);
end

== matlab function acc/relative_dynamic_estimated/Measurement_update_X1 ==
  data: X_e input; u input; X_b output
function X_b=fcn(X_e,u)
T=0.1;
F=[1 T 0.5*T^2;0 1 T;0 0 1];
G=[-1/6*T^3;-1/2*T^2;-T];

X_b=F*X_e+G*u;
end

== matlab function acc/Acceleration controller2 ==
  data: axc input; Tr output; Vxh input; Tb output; Rtotal output; m input
function [Tr,Tb,Rtotal]= fcn(axc, Vxh,m)
% m_hat = 1370+89.9+65.2+22*4; 
m_hat = m;
Cd_hat = 0.3;     %Aerodynamic Coefficient
fr_hat = 0.0038;  %Rolling Resistance Moment

zho = 1.206;  %Air Mass density
Af = 2.2; %Front Area
g = 9.81;
rw = 0.325; %Effective rolling radius 

% m_hat = 1/theta_hat(1);
% Cd_hat = theta_hat(2)*m_hat;
% fr_hat = theta_hat(3);

theta = 0;
% Resistance

Ra = 0.5*zho*Cd_hat*Af*Vxh^2;
Rg = m_hat*g*sin(theta);
Rr = fr_hat*m_hat*g*cos(theta);
Rtotal = (Ra + Rg + Rr)*rw;

% if Vxh<1
%     Ra=0;
%     Rg=0;
%     Rr=0;
%     Rtotal =0;
% else
%     Ra = 0.5*zho*Cd_hat*Af*Vxh^2;
%     Rg = m_hat*g*sin(theta);
%     Rr = fr_hat*m_hat*g*cos(theta);
%     Rtotal = (Ra + Rg + Rr)*rw;
% end

Tr = (m_hat*axc + Ra + Rg + Rr)*rw;
Tb = (m_hat*axc - Ra - Rg - Rr)*rw;

if axc >= 0
    Tr = Tr;
    Tb = 0;
else
    Tr = 0;
    Tb = Tb;
end

== matlab function acc/MATLAB Function3 ==
  data: Xf input; RR output; Yf input; Xh input; Yh input; RD output
function [RR,RD] = fcn(Xf,Yf,Xh,Yh)
RX=Xf-Xh;
RY=Yf-Yh;
if RX >= 0
    RR=sqrt(RX^2+RY^2);
    RD=atand(RY/RX);
else
    RR=sqrt(RX^2+RY^2);
    RD=atand(RY/RX)+180;
end
if RD < -0.1
    RD=RD+360;
end
end

== matlab function acc/Estimation_TTCy_PV ==
  data: R input; TTC1 output; V input; A input; TTC2 output
function [TTC1,TTC2] = TTCy(R,V,A)
TTCp1=10;
TTCp2=10;
if R < 0
    R=-R;
    V=-V;
    A=-A;
end
if R < 0.2 
   TTC1=0;
else
    if abs(A) > 1 && (V^2-2*A*R)>0
        TTCp1=(-V+sqrt(V^2-2*A*R))/A;
        TTCp2=(-V-sqrt(V^2-2*A*R))/A;
        if TTCp1>0 && TTCp2 >0
            TTC1 =min(TTCp1,TTCp2);
        elseif TTCp1 >= 0
            TTC1=TTCp1;
        else
            TTC1=TTCp2;
        end
    else
    TTC1=-R/V;
    end
end
if TTC1 > 5 
    TTC1=5;
end
if TTC1 < 0
    TTC1=5;
end

if R < 0.2 
   TTC2=0;
else
    TTC2=-R/V;
end

if TTC2 > 5
    TTC2=5;
end
if TTC2 < 0
    TTC2=5;
end
end

== matlab function acc/MATLAB Function17 ==
  data: trig input; u output; Yref input; tau input; Qs input; Rs input; steer_angle input; Vx input; Ax input
function u  = fcn( trig,Yref, tau, Qs,Rs,steer_angle,Vx,Ax)
%% parameter
Np=10;
Nc=3;
T = 0.1;

% if case1==1
%    Qs1=8;
%    Rs1=30;
%    Np=35;
% else
%    Qs1=6;
%    Rs1=1;
%    Np=35;
% end



if trig ==1


L=2.650;


Y_ref=Yref;


%% vehicle parameter

vx = ones(Np,1)*Vx; %10kph
%     vx=zeros(Np,1);
%     vx(1)=Vx;
%     for z=2:Np
%         vx(z)=vx(z-1)+Ax*T;
%     end
x_state = [0 0 steer_angle]';

%% Vehicle Kinematics Model
A  = [1 vx(1,1)*T vx(1,1)*T;
        0 1 vx(1,1)/L*T;
        0 0 -T/tau+1];
% ----------------------------------------%
% x = [y, yaw angle, steering wheel angle]
% state row =3, state column =3,
%-----------------------------------------%
sr =3;
sc =3;
B = [0 0 (1/tau)*T]';
H = [1 0 0]; % [1, sr]

%% MPC parameter
% ------------------------------------------------------------------------------------------%
% Am is a vertor [A(k); A(k+1); A(k+2) ... A(k+np-1)]
% ------------------------------------------------------------------------------------------%
Am = zeros(sr, sc, Np);
for i = 1 : Np
    Am(:, :, i) = [1 vx(i,1)*T vx(i,1)*T;
                    0 1 vx(i,1)/L*T;
                    0 0 -(T/tau)+1];
end
% ------------------------------------------------------------------------------------------%
% Amm is a vector [A(k); A(k)A(k+1); A(k)A(k+1)A(k+2) ... A(k+np-1)]
% ------------------------------------------------------------------------------------------%
Amm = zeros(sr, sc, Np);
Amm(:, :, 1) = Am(:, :, 1);
for i = 2 : Np
    Amm(:, :, i) = Am(:, :, i) * Amm(:, :, i - 1);
end
% ----------------------------------------------------------------------------------------------%
% F is a metric [H A(k); H A(k)A(k+1); H A(k)A(k+1)A(k+2) ... H A(k+np-1)]
% size = [np, sc]
% ----------------------------------------------------------------------------------------------%
F = zeros(Np, sc);
for i = 1 : Np
    F(i, :) = H * Amm(:, : ,i);
end

% ----------------------------------------------------------------------------------------------%
% K is a metric [H A(k); H A(k)A(k+1); H A(k)A(k+1)A(k+2) ... H A(k+np-1)]
%size = [np nc]
%[H*B                                 0             0  ...       0  ]
%[H*A(k)*B                       H*B          0  ...        0 ] 
%[H*A(k)*A(k+1)*B       H*A(k)*B      0  ...    H*B ]
% the following quation is modified

%[H*B                                 0                   0          0          ...           0 ]
%[H*A(k+1)*B                          H*B                 0          0          ...           0 ] 
%[H*A(k+2)*A(k+1)*B                 H*A(k+2)*B           H*B         0          ...           0 ]
%[H*A(k+3)*A(k+2)*A(k+1)*B        H*A(k+3)*A(k+2)*B     H*A(k+3)*B   H*B        ...           0 ]
%[H*A(k+np-1)*A(k+np-2)*...*A(k+np-np+1)*B      H*A(k+np-1)*A(k+np-2)*...*A(k+np-np+2)*B     H*A(k+3)*B   H*B        ...           0 ]
% ----------------------------------------------------------------------------------------------%
K = zeros(Np, Nc);
K(1,1) = H*B;
for i = 2 : Np
    K(i,1) = F(i-1, :) * B;
end
for i = 2 : Nc
    K(i : Np, i) = K(i - 1 : Np - 1, i - 1);
end

%% final K
% K = eye(Np, Np);
% K = K * (H*B);
% Kmm = zeros(sr, sc, Np, Np);
% for i = 2 : Np
%     
%     Kmm(:, :, i, i-1) = Am(:, :, i);
%     K(i, i-1) = H * Kmm(:, :, i, i-1) * B;
% end
% 
% r = 1;
% for i = 3 : Np
%     Kmm(:, :, i, 1) = Am(:, :, i) * Kmm(:, :, i-1, 1);
%     K(i, 1) = H * Kmm(:, :, i, 1) * B;
%     m = i;
%     while (m >= 4 && m<=Np)
%         Kmm(:, :, m, r) = Am(:, :, m) * Kmm(:, :, m-1, r);
%         K(m, r) = H * Kmm(:, :, m, r) * B;
%         m = m+1;
%     end
%     r = r+1;
% end
% 
% if Nc ~= Np
%     K = K (1:Np, 1:Nc);
% end

% K = zeros(Np, Nc);
% K(1,1) = H*B;
% for i = 2 : Np
% end

% ----------------------------------------------------------------------------------------------%
%Q is the weighting of reference error
%R is the weighting of control gain
%our object is the minimize the cost function between these two option
% ----------------------------------------------------------------------------------------------%

Q = eye(Np);

Q = Q * Qs;
R = eye(Nc);
R = R * Rs;

% ----------------------------------------------------------------------------------------------%
%cost function
%J = (Rs - Y) * Q * (Rs - Y)' + U * R * U'
% after differential the cost function,and let dJ=0, we can get
%U = inv(K' * Q * K + R) * K' * Q * (rs - F * x_state)
%solve U, and the vector U is the optimal control gain series 

%when Rs == 2
%J = (Rs1 - Y1) * Q1 * (Rs1 - Y1)' + (Rs2 - Y2) * Q2 * (Rs2 - Y2)' + U * R * U'
%U = inv(K1' * Q * K1 + K2' * Q * K2 + R) * (K1' * Q1 * (Rs1 - F1 * x_state) + K2' * Q2 * (Rs2 - F2 * x_state))
% ----------------------------------------------------------------------------------------------%

U = inv(K' * Q * K + R) * K' * Q * (Y_ref - F * x_state);
u=U(1);

else
    u=0;
end
end

== matlab function acc/Subsystem/longitudinal_driver_reference ==
  data: longitudinal_lane_refernce_trigger input; T input; Vxo input; Vxt input; ax_max input; jx_max input; Vx output; t output
function [Vx,t] = fcn(longitudinal_lane_refernce_trigger,T,Vxo,Vxt,ax_max,jx_max)
Vx=0;
Ax=0;
t=0;

if Vxt < Vxo
    ax_max=-ax_max;
    jx_max=-jx_max;
end

if longitudinal_lane_refernce_trigger==1

t1=ax_max/jx_max;
t2=(Vxt-Vxo)/ax_max;
t3=t1+t2;
t=T+0.1;


V1=Vxo+(0.5*jx_max*(t1^2));
V2=V1+(ax_max*(t2-t1));
   if t>=0 && t<=t1
       Ax=jx_max*t;
       Vx=double(Vxo+0.5*jx_max*(t^2));
   end
   if t>t1 && t<=t2
       Ax=ax_max;
       Vx=double(V1+(ax_max*(t-t1)));
   end
   if t>t2 && t<=t3
       Ax=ax_max-(jx_max*(t-t2));
       Vx=double(V2+ax_max*(t-t2)-0.5*jx_max*((t-t2)^2));
   end
   if t>t3
       Vx=double(Vxt);
       Ax=0;
   end
       

end
if longitudinal_lane_refernce_trigger==0
  Vx=double(Vxo);
 

   
end
end

== matlab function acc/Subsystem/longitudinal_driver_reference1 ==
  data: longitudinal_lane_refernce_trigger input; T input; Vxo input; Vxt input; ax_max input; jx_max input; Vx output; t output
function [Vx,t] = fcn(longitudinal_lane_refernce_trigger,T,Vxo,Vxt,ax_max,jx_max)
Vx=0;
Ax=0;
t=0;

if Vxt < Vxo
    ax_max=-ax_max;
    jx_max=-jx_max;
end

if longitudinal_lane_refernce_trigger==1

t1=ax_max/jx_max;
t2=(Vxt-Vxo)/ax_max;
t3=t1+t2;
t=T+0.1;


V1=Vxo+(0.5*jx_max*(t1^2));
V2=V1+(ax_max*(t2-t1));
   if t>=0 && t<=t1
       Ax=jx_max*t;
       Vx=double(Vxo+0.5*jx_max*(t^2));
   end
   if t>t1 && t<=t2
       Ax=ax_max;
       Vx=double(V1+(ax_max*(t-t1)));
   end
   if t>t2 && t<=t3
       Ax=ax_max-(jx_max*(t-t2));
       Vx=double(V2+ax_max*(t-t2)-0.5*jx_max*((t-t2)^2));
   end
   if t>t3
       Vx=double(Vxt);
       Ax=0;
   end
       

end
if longitudinal_lane_refernce_trigger==0
  Vx=double(Vxo);
 

   
end
end

== matlab function acc/Subsystem/longitudinal_driver_reference2 ==
  data: longitudinal_lane_refernce_trigger input; T input; Vxo input; Vxt input; ax_max input; jx_max input; Vx output; t output
function [Vx,t] = fcn(longitudinal_lane_refernce_trigger,T,Vxo,Vxt,ax_max,jx_max)
Vx=0;
Ax=0;
t=0;

if Vxt < Vxo
    ax_max=-ax_max;
    jx_max=-jx_max;
end

if longitudinal_lane_refernce_trigger==1

t1=ax_max/jx_max;
t2=(Vxt-Vxo)/ax_max;
t3=t1+t2;
t=T+0.1;


V1=Vxo+(0.5*jx_max*(t1^2));
V2=V1+(ax_max*(t2-t1));
   if t>=0 && t<=t1
       Ax=jx_max*t;
       Vx=double(Vxo+0.5*jx_max*(t^2));
   end
   if t>t1 && t<=t2
       Ax=ax_max;
       Vx=double(V1+(ax_max*(t-t1)));
   end
   if t>t2 && t<=t3
       Ax=ax_max-(jx_max*(t-t2));
       Vx=double(V2+ax_max*(t-t2)-0.5*jx_max*((t-t2)^2));
   end
   if t>t3
       Vx=double(Vxt);
       Ax=0;
   end
       

end
if longitudinal_lane_refernce_trigger==0
  Vx=double(Vxo);
 

   
end
end

== matlab function acc/Subsystem/longitudinal_driver_reference3 ==
  data: longitudinal_lane_refernce_trigger input; T input; Vxo input; Vxt input; ax_max input; jx_max input; Vx output; t output
function [Vx,t] = fcn(longitudinal_lane_refernce_trigger,T,Vxo,Vxt,ax_max,jx_max)
Vx=0;
Ax=0;
t=0;

if Vxt < Vxo
    ax_max=-ax_max;
    jx_max=-jx_max;
end

if longitudinal_lane_refernce_trigger==1

t1=ax_max/jx_max;
t2=(Vxt-Vxo)/ax_max;
t3=t1+t2;
t=T+0.1;


V1=Vxo+(0.5*jx_max*(t1^2));
V2=V1+(ax_max*(t2-t1));
   if t>=0 && t<=t1
       Ax=jx_max*t;
       Vx=double(Vxo+0.5*jx_max*(t^2));
   end
   if t>t1 && t<=t2
       Ax=ax_max;
       Vx=double(V1+(ax_max*(t-t1)));
   end
   if t>t2 && t<=t3
       Ax=ax_max-(jx_max*(t-t2));
       Vx=double(V2+ax_max*(t-t2)-0.5*jx_max*((t-t2)^2));
   end
   if t>t3
       Vx=double(Vxt);
       Ax=0;
   end
       

end
if longitudinal_lane_refernce_trigger==0
  Vx=double(Vxo);
 

   
end
end

== matlab function acc/Subsystem/longitudinal_driver_reference4 ==
  data: longitudinal_lane_refernce_trigger input; T input; Vxo input; Vxt input; ax_max input; jx_max input; Vx output; t output
function [Vx,t] = fcn(longitudinal_lane_refernce_trigger,T,Vxo,Vxt,ax_max,jx_max)
Vx=0;
Ax=0;
t=0;

if Vxt < Vxo
    ax_max=-ax_max;
    jx_max=-jx_max;
end

if longitudinal_lane_refernce_trigger==1

t1=ax_max/jx_max;
t2=(Vxt-Vxo)/ax_max;
t3=t1+t2;
t=T+0.1;


V1=Vxo+(0.5*jx_max*(t1^2));
V2=V1+(ax_max*(t2-t1));
   if t>=0 && t<=t1
       Ax=jx_max*t;
       Vx=double(Vxo+0.5*jx_max*(t^2));
   end
   if t>t1 && t<=t2
       Ax=ax_max;
       Vx=double(V1+(ax_max*(t-t1)));
   end
   if t>t2 && t<=t3
       Ax=ax_max-(jx_max*(t-t2));
       Vx=double(V2+ax_max*(t-t2)-0.5*jx_max*((t-t2)^2));
   end
   if t>t3
       Vx=double(Vxt);
       Ax=0;
   end
       

end
if longitudinal_lane_refernce_trigger==0
  Vx=double(Vxo);
 

   
end
end

== matlab function acc/Subsystem/longitudinal_driver_reference5 ==
  data: longitudinal_lane_refernce_trigger input; T input; Vxo input; Vxt input; ax_max input; jx_max input; Vx output; t output
function [Vx,t] = fcn(longitudinal_lane_refernce_trigger,T,Vxo,Vxt,ax_max,jx_max)
Vx=0;
Ax=0;
t=0;

if Vxt < Vxo
    ax_max=-ax_max;
    jx_max=-jx_max;
end

if longitudinal_lane_refernce_trigger==1

t1=ax_max/jx_max;
t2=(Vxt-Vxo)/ax_max;
t3=t1+t2;
t=T+0.1;


V1=Vxo+(0.5*jx_max*(t1^2));
V2=V1+(ax_max*(t2-t1));
   if t>=0 && t<=t1
       Ax=jx_max*t;
       Vx=double(Vxo+0.5*jx_max*(t^2));
   end
   if t>t1 && t<=t2
       Ax=ax_max;
       Vx=double(V1+(ax_max*(t-t1)));
   end
   if t>t2 && t<=t3
       Ax=ax_max-(jx_max*(t-t2));
       Vx=double(V2+ax_max*(t-t2)-0.5*jx_max*((t-t2)^2));
   end
   if t>t3
       Vx=double(Vxt);
       Ax=0;
   end
       

end
if longitudinal_lane_refernce_trigger==0
  Vx=double(Vxo);
 

   
end
end

== matlab function acc/Subsystem/longitudinal_driver_reference6 ==
  data: longitudinal_lane_refernce_trigger input; T input; Vxo input; Vxt input; ax_max input; jx_max input; Vx output; t output
function [Vx,t] = fcn(longitudinal_lane_refernce_trigger,T,Vxo,Vxt,ax_max,jx_max)
Vx=0;
Ax=0;
t=0;

if Vxt < Vxo
    ax_max=-ax_max;
    jx_max=-jx_max;
end

if longitudinal_lane_refernce_trigger==1

t1=ax_max/jx_max;
t2=(Vxt-Vxo)/ax_max;
t3=t1+t2;
t=T+0.1;


V1=Vxo+(0.5*jx_max*(t1^2));
V2=V1+(ax_max*(t2-t1));
   if t>=0 && t<=t1
       Ax=jx_max*t;
       Vx=double(Vxo+0.5*jx_max*(t^2));
   end
   if t>t1 && t<=t2
       Ax=ax_max;
       Vx=double(V1+(ax_max*(t-t1)));
   end
   if t>t2 && t<=t3
       Ax=ax_max-(jx_max*(t-t2));
       Vx=double(V2+ax_max*(t-t2)-0.5*jx_max*((t-t2)^2));
   end
   if t>t3
       Vx=double(Vxt);
       Ax=0;
   end
       

end
if longitudinal_lane_refernce_trigger==0
  Vx=double(Vxo);
 

   
end
end

== matlab function acc/relative_dynamic_estimated/Time_update_X1 ==
  data: Q input; R input; K output; M2 output; M input
function [K,M2] = fcn(Q,R,M)
T=0.1;
% Rw=1; %變速度
% R=0.0001;
% Rw=1; %定速80
% R=0.001;
F=[1 T 0.5*T^2;0 1 T;0 0 1];
H=[1 0 0];
G=[-(T^3)/6;-(T^2)/2;-T];
G2=[(T^3)/6;(T^2)/2;T];

P=M-M*H'*inv(H*M*H'+R)*H*M;
M2=F*P*F'+G2*Q*G2';
% M2=F*P*F'+Q;
K=P*H'*inv(R);
end

== matlab function acc/relative_dynamic_estimated/MATLAB Function1 ==
  data: X_b input; X_e output; K input; y input; d output; e output
function [X_e,d,e] = fcn(X_b,K,y)
H=[1 0 0];
d=y-H*X_b;
X_e=X_b+K*(y-H*X_b);
e=y-H*X_e;
end

== matlab function acc/relative_dynamic_estimated/MATLAB Function2 ==
  data: Q input; Q2 output; R input; M input; e input; d input; K input; R2 output; G output
function [Q2,R2,G] = fcn(Q,R,M,e,d,K)
a=1;
b=1;
H=[1 0 0];
R2=a*R+(1-a)*(e*e'+H*M*H');

Q2=b*Q+2*(1-b)*(K*d*d'*K');
G=0*Q+K*d*d*K';
end
